simulink model "ControleFF_D_NL"  (R2020b)
settings: Solver=FixedStepAuto  StartTime=0  StopTime=10  FixedStep=1e-3  RelTol=1e-3
values from neighbouring files (symbols this model uses):
  alpha = alpha_vec(l)    [kermani_parameters.m]    (also in teste_controle_nao_linear.m = 1.25)
  Beff = 1    [kermani_parameters.m]    (also in teste_controle_nao_linear.m = 50)
  Fc = Fc_vec(k)    [kermani_parameters.m]    (also in teste_controle_nao_linear.m = 2173.5)
  Fs = Fs_vec(j)    [kermani_parameters.m]    (also in teste_controle_nao_linear.m = 2673.5)
  Jeff = 0.5    [kermani_parameters.m]    (also in teste_controle_nao_linear.m)
  K = (90/12)*(2*pi/60)    (= 0.785398163397)    [kermani_parameters.m]    (also in teste_controle_nao_linear.m)
  Kd = (2*xi*wn*Jeff - Beff)/K    (= 17.8253536263)    [kermani_parameters.m]    (also in teste_controle_nao_linear.m = -44.5633840657)
  Kp = (wn^2*Jeff)/K    (= 143.239448783)    [kermani_parameters.m]    (also in teste_controle_nao_linear.m)
  N = 3    [kermani_parameters.m]    (also in teste_controle_nao_linear.m)
  phi = 43.47    [teste_controle_nao_linear.m]
  r = 1./[231.22*4 139.138 139.138 231.22 231.22]    [kermani_parameters.m]    (also in teste_controle_nao_linear.m)
  sigma0 = sigma0_vec(m)    [kermani_parameters.m]    (also in teste_controle_nao_linear.m = 10000)
  sigma1 = sigma1_vec(n)    [kermani_parameters.m]    (also in teste_controle_nao_linear.m = 1000)
  sigma2 = sigma2_vec(o)    [kermani_parameters.m]    (also in teste_controle_nao_linear.m = 10)
libraries: simulink_extras x21
(part 1 of 14)
settings Model: Creator=Karoline  LastModifiedBy=lunet
settings DataIOCC: ReturnWorkspaceOutputs=off
settings DebuggingCC: ArithmeticOperatorsInVariantConditions=warning
settings SFSimCC: SimUseLocalCustomCode=off  CustomCodeUndefinedFunction=UseInterfaceOnly
settings RTWCC: RTWUseLocalCustomCode=off
settings CodeAppCC: StateflowObjectComments=on

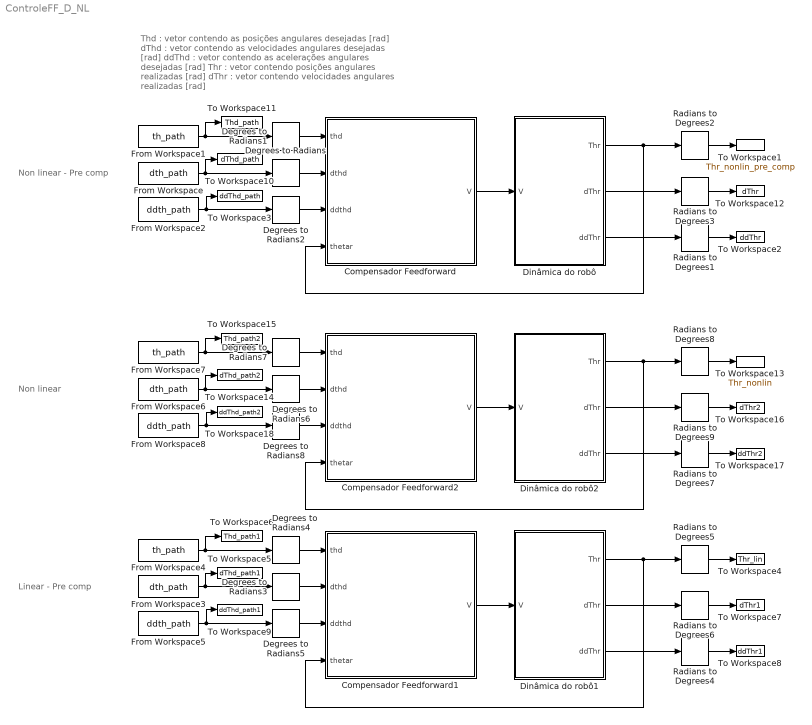
== system ControleFF_D_NL ==
  note: Non linear - Pre comp
  note: Thd : vetor contendo as posições angulares desejadas [rad]
      | dThd : vetor contendo as velocidades angulares desejadas [rad]
      | ddThd : vetor contendo as acelerações angulares desejadas [rad]
      |
      | Thr : vetor contendo posições angulares realizadas [rad]
      | dThr : vetor contendo velocidades angulares realizadas [rad]
  note: Non linear
  note: Linear - Pre comp
  Compensador Feedforward : Subsystem
  Compensador Feedforward1 : Subsystem
  Compensador Feedforward2 : Subsystem
  Degrees to Radians{,1..8} (9 alike) : simulink_extras/Transformations/Degrees to Radians
  Dinâmica do robô : Subsystem
  Dinâmica do robô1 : Subsystem
  Dinâmica do robô2 : Subsystem
  From Workspace : FromWorkspace  VariableName=dth_path
  From Workspace1 : FromWorkspace  VariableName=th_path
  From Workspace2 : FromWorkspace  VariableName=ddth_path
  From Workspace3 : FromWorkspace  VariableName=dth_path
  From Workspace4 : FromWorkspace  VariableName=th_path
  From Workspace5 : FromWorkspace  VariableName=ddth_path
  From Workspace6 : FromWorkspace  VariableName=dth_path
  From Workspace7 : FromWorkspace  VariableName=th_path
  From Workspace8 : FromWorkspace  VariableName=ddth_path
  Radians to Degrees{1..9} (9 alike) : simulink_extras/Transformations/Radians to Degrees
  To Workspace1 : ToWorkspace  VariableName=Thr_nonlin_pre_comp  SaveFormat=Structure With Time  SampleTime=-1
  To Workspace10 : ToWorkspace  VariableName=dThd_path  SaveFormat=Structure With Time  SampleTime=-1
  To Workspace11 : ToWorkspace  VariableName=Thd_path  SaveFormat=Structure With Time  SampleTime=-1
  To Workspace12 : ToWorkspace  VariableName=dThr  SaveFormat=Structure With Time  SampleTime=-1
  To Workspace13 : ToWorkspace  VariableName=Thr_nonlin  SaveFormat=Structure With Time  SampleTime=-1
  To Workspace14 : ToWorkspace  VariableName=dThd_path2  SaveFormat=Structure With Time  SampleTime=-1
  To Workspace15 : ToWorkspace  VariableName=Thd_path2  SaveFormat=Structure With Time  SampleTime=-1
  To Workspace16 : ToWorkspace  VariableName=dThr2  SaveFormat=Structure With Time  SampleTime=-1
  To Workspace17 : ToWorkspace  VariableName=ddThr2  SaveFormat=Structure With Time  SampleTime=-1
  To Workspace18 : ToWorkspace  VariableName=ddThd_path2  SaveFormat=Structure With Time  SampleTime=-1
  To Workspace2 : ToWorkspace  VariableName=ddThr  SaveFormat=Structure With Time  SampleTime=-1
  To Workspace3 : ToWorkspace  VariableName=ddThd_path  SaveFormat=Structure With Time  SampleTime=-1
  To Workspace4 : ToWorkspace  VariableName=Thr_lin  SaveFormat=Structure With Time  SampleTime=-1
  To Workspace5 : ToWorkspace  VariableName=dThd_path1  SaveFormat=Structure With Time  SampleTime=-1
  To Workspace6 : ToWorkspace  VariableName=Thd_path1  SaveFormat=Structure With Time  SampleTime=-1
  To Workspace7 : ToWorkspace  VariableName=dThr1  SaveFormat=Structure With Time  SampleTime=-1
  To Workspace8 : ToWorkspace  VariableName=ddThr1  SaveFormat=Structure With Time  SampleTime=-1
  To Workspace9 : ToWorkspace  VariableName=ddThd_path1  SaveFormat=Structure With Time  SampleTime=-1
  wires:
  Dinâmica do robô/2("dThr ") -> Radians to Degrees3/1
  Compensador Feedforward/1(V) -> Dinâmica do robô/1(V)
  Dinâmica do robô/1(Thr) -> Compensador Feedforward/4(thetar), Radians to Degrees2/1
  From Workspace2/1 -> To Workspace3/1, Degrees to Radians2/1
  Degrees to Radians2/1 -> Compensador Feedforward/3(ddthd)
  From Workspace/1 -> Degrees to Radians/1, To Workspace10/1
  From Workspace1/1 -> Degrees to Radians1/1, To Workspace11/1
  Degrees to Radians1/1 -> Compensador Feedforward/1(thd)
  Degrees to Radians/1 -> Compensador Feedforward/2(dthd)
  Radians to Degrees3/1 -> To Workspace12/1
  Radians to Degrees2/1 -> To Workspace1/1
  Radians to Degrees1/1 -> To Workspace2/1
  Dinâmica do robô/3(ddThr) -> Radians to Degrees1/1
  Degrees to Radians3/1 -> Compensador Feedforward1/2(dthd)
  Radians to Degrees6/1 -> To Workspace7/1
  Radians to Degrees5/1 -> To Workspace4/1
  Radians to Degrees4/1 -> To Workspace8/1
  Dinâmica do robô1/3(ddThr) -> Radians to Degrees4/1
  From Workspace3/1 -> Degrees to Radians3/1, To Workspace5/1
  Dinâmica do robô1/1(Thr) -> Compensador Feedforward1/4(thetar), Radians to Degrees5/1
  From Workspace5/1 -> To Workspace9/1, Degrees to Radians5/1
  From Workspace4/1 -> Degrees to Radians4/1, To Workspace6/1
  Compensador Feedforward1/1(V) -> Dinâmica do robô1/1(V)
  Degrees to Radians5/1 -> Compensador Feedforward1/3(ddthd)
  Degrees to Radians4/1 -> Compensador Feedforward1/1(thd)
  Dinâmica do robô1/2("dThr ") -> Radians to Degrees6/1
  Degrees to Radians6/1 -> Compensador Feedforward2/2(dthd)
  Radians to Degrees9/1 -> To Workspace16/1
  Radians to Degrees8/1 -> To Workspace13/1
  Radians to Degrees7/1 -> To Workspace17/1
  Dinâmica do robô2/3(ddThr) -> Radians to Degrees7/1
  From Workspace6/1 -> Degrees to Radians6/1, To Workspace14/1
  Dinâmica do robô2/1(Thr) -> Compensador Feedforward2/4(thetar), Radians to Degrees8/1
  From Workspace8/1 -> To Workspace18/1, Degrees to Radians8/1
  From Workspace7/1 -> Degrees to Radians7/1, To Workspace15/1
  Compensador Feedforward2/1(V) -> Dinâmica do robô2/1(V)
  Degrees to Radians8/1 -> Compensador Feedforward2/3(ddthd)
  Degrees to Radians7/1 -> Compensador Feedforward2/1(thd)
  Dinâmica do robô2/2("dThr ") -> Radians to Degrees9/1

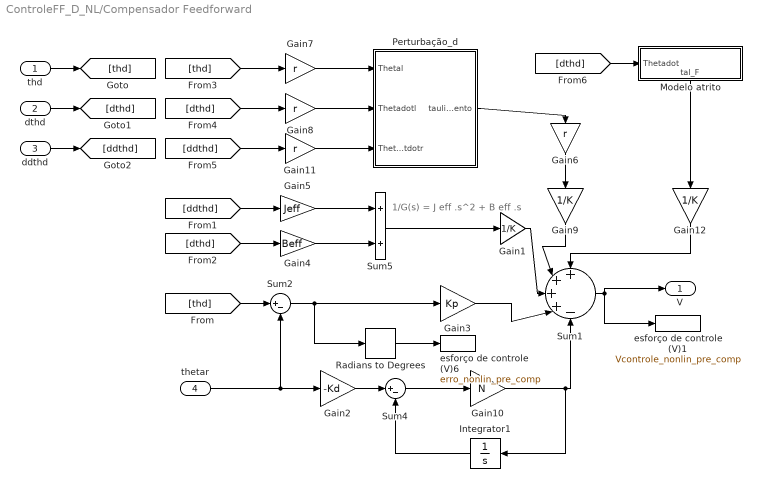
== system ControleFF_D_NL/Compensador Feedforward ==
  note: 1/G(s) = J eff .s^2 + B eff .s
  thd : Inport
  dthd : Inport  Port=2
  ddthd : Inport  Port=3
  thetar : Inport  Port=4
  Gain1 : Gain  Gain=1/K
  Gain10 : Gain  Gain=N
  Gain{6..8,11} (4 alike) : Gain  Gain=r
  Gain12 : Gain  Gain=1/K
  Gain2 : Gain  Gain=-Kd
  Gain3 : Gain  Gain=Kp
  Gain4 : Gain  Gain=Beff
  Gain5 : Gain  Gain=Jeff
  Gain9 : Gain  Gain=1/K
  Integrator1 : Integrator
  Modelo atrito : Subsystem
      settings: PortSchema="{\"entries\":[{\"content\":{\"sides\":[{\"content\":{\"connectorIds\":[\"In1\"]},\"type\":\"ConnectorPlacement.EquallySpacedRectSide\",\"uuid\":\"4cdf76dd-7842-4f53-aa61-23d67f277515\"},{\"content\":{\"connectorIds\":[],\"side\":\"RIGHT\"},\"type\":\"ConnectorPlacement.EquallySpacedRectSide\",\"uuid\":\"e76865b0-8d89-469f-9903-74c23d9bc715\"},{\"content\":{\"connectorIds\":[],\"side\":\"TOP\"},\"type\":\"ConnectorPlacement.EquallySpacedRectSide\",\"uuid\":\"84af05c2-3cf0-417f-8bc5-33473f29c4a4\"},{\"content\":{\"connectorIds\":[\"Out1\"],\"side\":\"BOTTOM\"},\"type\":\"ConnectorPlacement.EquallySpacedRectSide\",\"uuid\":\"8432edb9-61b6-48e7-b184-4a420fe1e6b9\"},{\"content\":{\"connectorIds\":[],\"side\":\"HIDDEN\"},\"type\":\"ConnectorPlacement.EquallySpacedRectSide\",\"uuid\":\"b24fdc73-1a64-48d6-a255-97fbfad7318c\"}]},\"type\":\"ConnectorPlacement.EquallySpacedConnector\",\"uuid\":\"378be7c8-9b7c-4aa3-9a72-c75578af889e\"}],\"packageUris\":[\"http://schema.mathworks.com/mf0/Connector/R2020b\"],\"version\":\"1.0\"}"
  Perturbação_d : Subsystem
  Radians to Degrees : simulink_extras/Transformations/Radians to Degrees
  Sum1 : Sum  Inputs=+|+|+|+|-
  Sum2 : Sum  Inputs=|+-
  Sum4 : Sum  Inputs=|+-
  Sum5 : Sum
  esforço de controle (V)1 : ToWorkspace  VariableName=Vcontrole_nonlin_pre_comp  SaveFormat=Structure With Time  SampleTime=-1
  esforço de controle (V)6 : ToWorkspace  VariableName=erro_nonlin_pre_comp  SaveFormat=Structure With Time  SampleTime=-1
  V : Outport  VectorParamsAs1DForOutWhenUnconnected=off
  wires:
  Gain2/1 -> Sum4/1
  thetar/1 -> Sum2/2, Gain2/1
  Sum4/1 -> Gain10/1
  Integrator1/1 -> Sum4/2
  Gain10/1 -> Sum1/5, Integrator1/1
  Gain4/1 -> Sum5/2
  Gain5/1 -> Sum5/1
  Sum5/1 -> Gain1/1
  Gain8/1 -> Perturbação_d/2(Thetadotl)
  Gain7/1 -> Perturbação_d/1(Thetal)
  [thd] -> Gain7/1
  [dthd] -> Gain8/1
  Perturbação_d/1(tauligamento) -> Gain6/1
  Gain6/1 -> Gain9/1
  Gain9/1 -> Sum1/2
  thd/1 -> [thd]
  [thd] -> Sum2/1
  ddthd/1 -> [ddthd]
  [ddthd] -> Gain5/1
  dthd/1 -> [dthd]
  [dthd] -> Gain4/1
  Gain3/1 -> Sum1/4
  Gain1/1 -> Sum1/3
  Sum1/1 -> V/1, esforço de controle (V)1/1
  Radians to Degrees/1 -> esforço de controle (V)6/1
  Sum2/1 -> Radians to Degrees/1, Gain3/1
  [ddthd] -> Gain11/1
  Gain11/1 -> Perturbação_d/3(Thetadotdotr)
  [dthd] -> Modelo atrito/1(Thetadot)
  Modelo atrito/1(tal_F) -> Gain12/1
  Gain12/1 -> Sum1/1

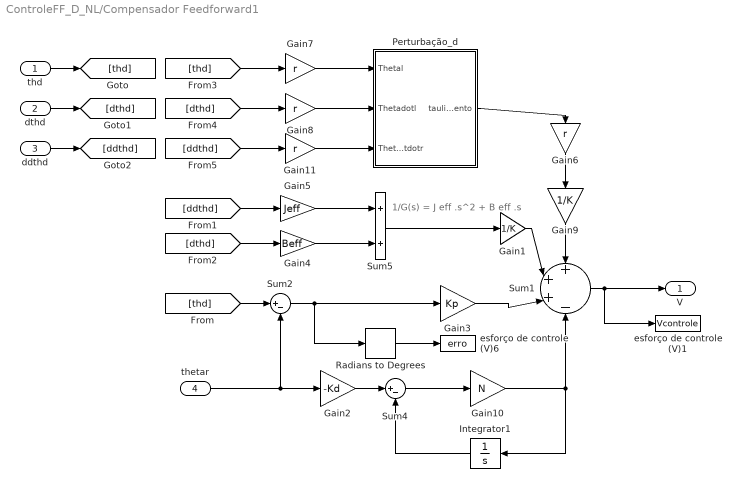
== system ControleFF_D_NL/Compensador Feedforward1 ==
  note: 1/G(s) = J eff .s^2 + B eff .s
  thd : Inport
  dthd : Inport  Port=2
  ddthd : Inport  Port=3
  thetar : Inport  Port=4
  Gain1 : Gain  Gain=1/K
  Gain10 : Gain  Gain=N
  Gain{6..8,11} (4 alike) : Gain  Gain=r
  Gain2 : Gain  Gain=-Kd
  Gain3 : Gain  Gain=Kp
  Gain4 : Gain  Gain=Beff
  Gain5 : Gain  Gain=Jeff
  Gain9 : Gain  Gain=1/K
  Integrator1 : Integrator
  Perturbação_d : Subsystem
  Radians to Degrees : simulink_extras/Transformations/Radians to Degrees
  Sum1 : Sum  Inputs=+|+|+|-
  Sum2 : Sum  Inputs=|+-
  Sum4 : Sum  Inputs=|+-
  Sum5 : Sum
  esforço de controle (V)1 : ToWorkspace  VariableName=Vcontrole  SaveFormat=Structure With Time  SampleTime=-1
  esforço de controle (V)6 : ToWorkspace  VariableName=erro  SaveFormat=Structure With Time  SampleTime=-1
  V : Outport  VectorParamsAs1DForOutWhenUnconnected=off
  wires:
  Gain2/1 -> Sum4/1
  thetar/1 -> Sum2/2, Gain2/1
  Sum4/1 -> Gain10/1
  Integrator1/1 -> Sum4/2
  Gain10/1 -> Sum1/4, Integrator1/1
  Gain4/1 -> Sum5/2
  Gain5/1 -> Sum5/1
  Sum5/1 -> Gain1/1
  Gain8/1 -> Perturbação_d/2(Thetadotl)
  Gain7/1 -> Perturbação_d/1(Thetal)
  [thd] -> Gain7/1
  [dthd] -> Gain8/1
  Perturbação_d/1(tauligamento) -> Gain6/1
  Gain6/1 -> Gain9/1
  Gain9/1 -> Sum1/1
  thd/1 -> [thd]
  [thd] -> Sum2/1
  ddthd/1 -> [ddthd]
  [ddthd] -> Gain5/1
  dthd/1 -> [dthd]
  [dthd] -> Gain4/1
  Gain3/1 -> Sum1/3
  Gain1/1 -> Sum1/2
  Sum1/1 -> esforço de controle (V)1/1, V/1
  Radians to Degrees/1 -> esforço de controle (V)6/1
  Sum2/1 -> Radians to Degrees/1, Gain3/1
  [ddthd] -> Gain11/1
  Gain11/1 -> Perturbação_d/3(Thetadotdotr)

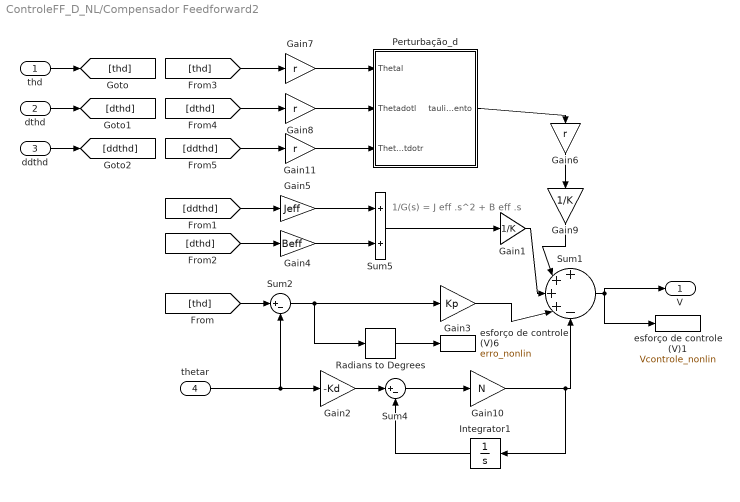
== system ControleFF_D_NL/Compensador Feedforward2 ==
  note: 1/G(s) = J eff .s^2 + B eff .s
  thd : Inport
  dthd : Inport  Port=2
  ddthd : Inport  Port=3
  thetar : Inport  Port=4
  Gain1 : Gain  Gain=1/K
  Gain10 : Gain  Gain=N
  Gain{6..8,11} (4 alike) : Gain  Gain=r
  Gain2 : Gain  Gain=-Kd
  Gain3 : Gain  Gain=Kp
  Gain4 : Gain  Gain=Beff
  Gain5 : Gain  Gain=Jeff
  Gain9 : Gain  Gain=1/K
  Integrator1 : Integrator
  Perturbação_d : Subsystem
  Radians to Degrees : simulink_extras/Transformations/Radians to Degrees
  Sum1 : Sum  Inputs=+|+|+|+|-
  Sum2 : Sum  Inputs=|+-
  Sum4 : Sum  Inputs=|+-
  Sum5 : Sum
  esforço de controle (V)1 : ToWorkspace  VariableName=Vcontrole_nonlin  SaveFormat=Structure With Time  SampleTime=-1
  esforço de controle (V)6 : ToWorkspace  VariableName=erro_nonlin  SaveFormat=Structure With Time  SampleTime=-1
  V : Outport  VectorParamsAs1DForOutWhenUnconnected=off
  wires:
  Gain2/1 -> Sum4/1
  thetar/1 -> Sum2/2, Gain2/1
  Sum4/1 -> Gain10/1
  Integrator1/1 -> Sum4/2
  Gain10/1 -> Sum1/5, Integrator1/1
  Gain4/1 -> Sum5/2
  Gain5/1 -> Sum5/1
  Sum5/1 -> Gain1/1
  Gain8/1 -> Perturbação_d/2(Thetadotl)
  Gain7/1 -> Perturbação_d/1(Thetal)
  [thd] -> Gain7/1
  [dthd] -> Gain8/1
  Perturbação_d/1(tauligamento) -> Gain6/1
  Gain6/1 -> Gain9/1
  Gain9/1 -> Sum1/2
  thd/1 -> [thd]
  [thd] -> Sum2/1
  ddthd/1 -> [ddthd]
  [ddthd] -> Gain5/1
  dthd/1 -> [dthd]
  [dthd] -> Gain4/1
  Gain3/1 -> Sum1/4
  Gain1/1 -> Sum1/3
  Sum1/1 -> V/1, esforço de controle (V)1/1
  Radians to Degrees/1 -> esforço de controle (V)6/1
  Sum2/1 -> Radians to Degrees/1, Gain3/1
  [ddthd] -> Gain11/1
  Gain11/1 -> Perturbação_d/3(Thetadotdotr)

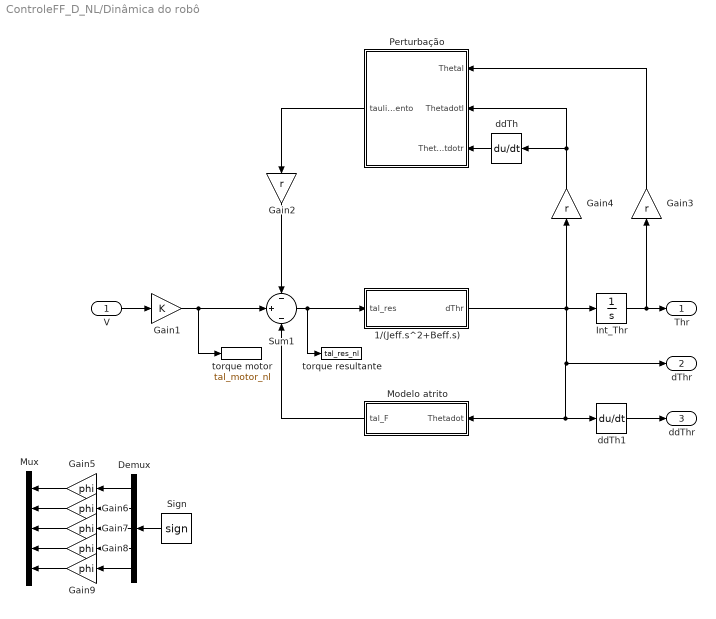
== system ControleFF_D_NL/Dinâmica do robô ==
  V : Inport
  1/(Jeff.s^2+Beff.s) : Subsystem
  Demux : Demux  Outputs=5
  Gain1 : Gain  Gain=K
  Gain2 : Gain  Gain=r
  Gain3 : Gain  Gain=r
  Gain4 : Gain  Gain=r
  Gain{5..9} (5 alike) : Gain  Gain=phi
  Int_Thr : Integrator  Tag=Int_Thr  InitialCondition=[0 0 0 0 0]
  Modelo atrito : Subsystem
  Mux : Mux  Inputs=5
  Perturbação : Subsystem
  Sign : Signum
  Sum1 : Sum  Inputs=-|+|-
  ddTh : Derivative
  ddTh1 : Derivative
  torque motor : ToWorkspace  VariableName=tal_motor_nl  SaveFormat=Structure With Time  SampleTime=-1
  torque resultante : ToWorkspace  VariableName=tal_res_nl  SaveFormat=Structure With Time  SampleTime=-1
  Thr : Outport  VectorParamsAs1DForOutWhenUnconnected=off
  "dThr " : Outport  Port=2  VectorParamsAs1DForOutWhenUnconnected=off
  ddThr : Outport  Port=3  VectorParamsAs1DForOutWhenUnconnected=off
  wires:
  Perturbação/1(tauligamento) -> Gain2/1
  Gain1/1 -> torque motor/1, Sum1/2
  Int_Thr/1 -> Thr/1, Gain3/1
  V/1 -> Gain1/1
  Gain2/1 -> Sum1/1
  ddTh/1 -> Perturbação/3(Thetadotdotr)
  Gain3/1 -> Perturbação/1(Thetal)
  Gain4/1 -> ddTh/1, Perturbação/2(Thetadotl)
  Sum1/1 -> torque resultante/1, 1/(Jeff.s^2+Beff.s)/1(tal_res)
  ddTh1/1 -> ddThr/1
  Sign/1 -> Demux/1
  Demux/1 -> Gain5/1
  Gain5/1 -> Mux/1
  Demux/2 -> Gain6/1
  Demux/3 -> Gain7/1
  Demux/4 -> Gain8/1
  Demux/5 -> Gain9/1
  Gain6/1 -> Mux/2
  Gain7/1 -> Mux/3
  Gain8/1 -> Mux/4
  Gain9/1 -> Mux/5
  1/(Jeff.s^2+Beff.s)/1(dThr) -> Modelo atrito/1(Thetadot), ddTh1/1, "dThr "/1, Gain4/1, Int_Thr/1
  Modelo atrito/1(tal_F) -> Sum1/3

== system ControleFF_D_NL/Dinâmica do robô1 ==
  V : Inport
  1/(Jeff.s^2+Beff.s) : Subsystem
  Demux : Demux  Outputs=5
  Gain1 : Gain  Gain=K
  Gain2 : Gain  Gain=r
  Gain3 : Gain  Gain=r
  Gain4 : Gain  Gain=r
  Gain{5..9} (5 alike) : Gain  Gain=phi
  Int_Thr : Integrator  Tag=Int_Thr  InitialCondition=[0 0 0 0 0]
  Mux : Mux  Inputs=5
  Perturbação : Subsystem
  Scope1 : Scope
  Sign : Signum
  Sum1 : Sum  Inputs=-+|
  ddTh : Derivative
  ddTh1 : Derivative
  torque motor : ToWorkspace  VariableName=tal_motor  SaveFormat=Structure With Time  SampleTime=-1
  torque resultante : ToWorkspace  VariableName=tal_res  SaveFormat=Structure With Time  SampleTime=-1
  Thr : Outport  VectorParamsAs1DForOutWhenUnconnected=off
  "dThr " : Outport  Port=2  VectorParamsAs1DForOutWhenUnconnected=off
  ddThr : Outport  Port=3  VectorParamsAs1DForOutWhenUnconnected=off
  wires:
  Perturbação/1(tauligamento) -> Gain2/1
  Gain1/1 -> torque motor/1, Sum1/2
  Int_Thr/1 -> Thr/1, Scope1/1, Gain3/1
  V/1 -> Gain1/1
  Gain2/1 -> Sum1/1
  ddTh/1 -> Perturbação/3(Thetadotdotr)
  Gain3/1 -> Perturbação/1(Thetal)
  Gain4/1 -> ddTh/1, Perturbação/2(Thetadotl)
  Sum1/1 -> torque resultante/1, 1/(Jeff.s^2+Beff.s)/1(tal_res)
  ddTh1/1 -> ddThr/1
  Sign/1 -> Demux/1
  Demux/1 -> Gain5/1
  Gain5/1 -> Mux/1
  Demux/2 -> Gain6/1
  Demux/3 -> Gain7/1
  Demux/4 -> Gain8/1
  Demux/5 -> Gain9/1
  Gain6/1 -> Mux/2
  Gain7/1 -> Mux/3
  Gain8/1 -> Mux/4
  Gain9/1 -> Mux/5
  1/(Jeff.s^2+Beff.s)/1(dThr) -> ddTh1/1, "dThr "/1, Gain4/1, Int_Thr/1

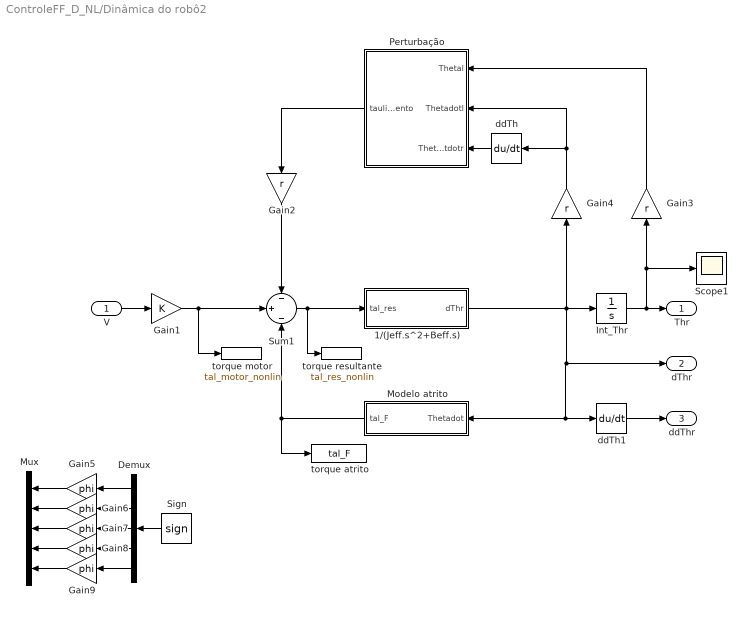
== system ControleFF_D_NL/Dinâmica do robô2 ==
  V : Inport
  1/(Jeff.s^2+Beff.s) : Subsystem
  Demux : Demux  Outputs=5
  Gain1 : Gain  Gain=K
  Gain2 : Gain  Gain=r
  Gain3 : Gain  Gain=r
  Gain4 : Gain  Gain=r
  Gain{5..9} (5 alike) : Gain  Gain=phi
  Int_Thr : Integrator  Tag=Int_Thr  InitialCondition=[0 0 0 0 0]
  Modelo atrito : Subsystem
  Mux : Mux  Inputs=5
  Perturbação : Subsystem
  Scope1 : Scope
  Sign : Signum
  Sum1 : Sum  Inputs=-|+|-
  ddTh : Derivative
  ddTh1 : Derivative
  torque atrito : ToWorkspace  VariableName=tal_F  SaveFormat=Structure With Time  SampleTime=-1
  torque motor : ToWorkspace  VariableName=tal_motor_nonlin  SaveFormat=Structure With Time  SampleTime=-1
  torque resultante : ToWorkspace  VariableName=tal_res_nonlin  SaveFormat=Structure With Time  SampleTime=-1
  Thr : Outport  VectorParamsAs1DForOutWhenUnconnected=off
  "dThr " : Outport  Port=2  VectorParamsAs1DForOutWhenUnconnected=off
  ddThr : Outport  Port=3  VectorParamsAs1DForOutWhenUnconnected=off
  wires:
  Perturbação/1(tauligamento) -> Gain2/1
  Gain1/1 -> torque motor/1, Sum1/2
  Int_Thr/1 -> Thr/1, Scope1/1, Gain3/1
  V/1 -> Gain1/1
  Gain2/1 -> Sum1/1
  ddTh/1 -> Perturbação/3(Thetadotdotr)
  Gain3/1 -> Perturbação/1(Thetal)
  Gain4/1 -> ddTh/1, Perturbação/2(Thetadotl)
  Sum1/1 -> torque resultante/1, 1/(Jeff.s^2+Beff.s)/1(tal_res)
  ddTh1/1 -> ddThr/1
  Sign/1 -> Demux/1
  Demux/1 -> Gain5/1
  Gain5/1 -> Mux/1
  Demux/2 -> Gain6/1
  Demux/3 -> Gain7/1
  Demux/4 -> Gain8/1
  Demux/5 -> Gain9/1
  Gain6/1 -> Mux/2
  Gain7/1 -> Mux/3
  Gain8/1 -> Mux/4
  Gain9/1 -> Mux/5
  1/(Jeff.s^2+Beff.s)/1(dThr) -> Modelo atrito/1(Thetadot), ddTh1/1, "dThr "/1, Gain4/1, Int_Thr/1
  Modelo atrito/1(tal_F) -> Sum1/3, torque atrito/1

== system ControleFF_D_NL/Compensador Feedforward/Modelo atrito ==
  note: z
  note: zdot
  Thetadot : Inport
  Abs : Abs
  Add : Sum  Inputs=+++
  Divide : Product  Inputs=*/*
  Integrator : Integrator
  Sigma0 : Gain  Gain=sigma0
  Sigma1 : Gain  Gain=sigma1
  Sigma2 : Gain  Gain=sigma2
  Sum : Sum  Inputs=|+-
  s_Thetadot : Subsystem
      settings: PortSchema="{\"entries\":[{\"content\":{\"sides\":[{\"content\":{\"connectorIds\":[]},\"type\":\"ConnectorPlacement.EquallySpacedRectSide\",\"uuid\":\"4c4b190b-c928-4253-93d1-fd2ae137e0ab\"},{\"content\":{\"connectorIds\":[\"Out1\"],\"side\":\"RIGHT\"},\"type\":\"ConnectorPlacement.EquallySpacedRectSide\",\"uuid\":\"6a4109ad-b0a7-44dc-94f8-84112378c3da\"},{\"content\":{\"connectorIds\":[\"In1\"],\"side\":\"TOP\"},\"type\":\"ConnectorPlacement.EquallySpacedRectSide\",\"uuid\":\"364d9b06-17df-4fa5-ae25-87ed6816814d\"},{\"content\":{\"connectorIds\":[],\"side\":\"HIDDEN\"},\"type\":\"ConnectorPlacement.EquallySpacedRectSide\",\"uuid\":\"e93aa933-b8be-40f2-a8c0-ee27516241e6\"}]},\"type\":\"ConnectorPlacement.EquallySpacedConnector\",\"uuid\":\"c598e9c2-b687-45ab-b3d0-f2b281a49fb7\"}],\"packageUris\":[\"http://schema.mathworks.com/mf0/Connector/R2020b\"],\"version\":\"1.0\"}"
  tal_F : Outport
  wires:
  Sigma0/1 -> Divide/3, Add/3
  Sigma1/1 -> Add/2
  Divide/1 -> Sum/2
  Abs/1 -> s_Thetadot/1(|Thetadot|), Divide/1
  s_Thetadot/1(s_Thetadot) -> Divide/2
  Sum/1 -> Sigma1/1, Integrator/1
  Thetadot/1 -> Sigma2/1, Sum/1, Abs/1
  Sigma2/1 -> Add/1
  Integrator/1 -> Sigma0/1
  Add/1 -> tal_F/1

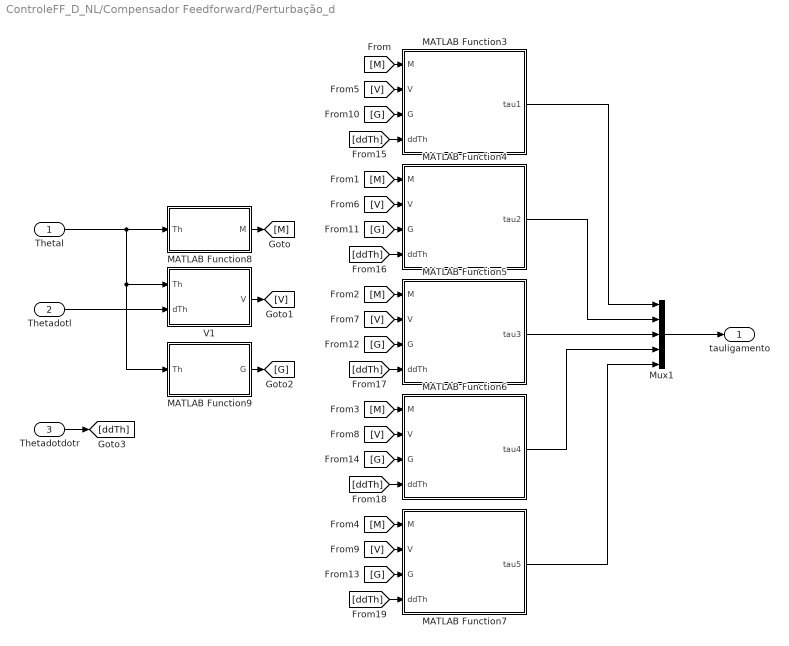
== system ControleFF_D_NL/Compensador Feedforward/Perturbação_d ==
  Thetal : Inport
  Thetadotl : Inport  Port=2
  Thetadotdotr : Inport  Port=3
  MATLAB Function3 : MATLAB Function  TreatAsAtomicUnit=on
  MATLAB Function4 : MATLAB Function  TreatAsAtomicUnit=on
  MATLAB Function5 : MATLAB Function  TreatAsAtomicUnit=on
  MATLAB Function6 : MATLAB Function  TreatAsAtomicUnit=on
  MATLAB Function7 : MATLAB Function  TreatAsAtomicUnit=on
  MATLAB Function8 : MATLAB Function  TreatAsAtomicUnit=on
  MATLAB Function9 : MATLAB Function  TreatAsAtomicUnit=on
  Mux1 : Mux  Inputs=5
  V1 : MATLAB Function  TreatAsAtomicUnit=on
  tauligamento : Outport  VectorParamsAs1DForOutWhenUnconnected=off
  wires:
  [G] -> MATLAB Function6/3(G)
  MATLAB Function8/1(M) -> [M]
  [M] -> MATLAB Function6/1(M)
  [M] -> MATLAB Function4/1(M)
  [M] -> MATLAB Function3/1(M)
  Thetal/1 -> MATLAB Function8/1(Th), MATLAB Function9/1(Th), V1/1(Th)
  [ddTh] -> MATLAB Function5/4(ddTh)
  [V] -> MATLAB Function3/2(V)
  [ddTh] -> MATLAB Function3/4(ddTh)
  [G] -> MATLAB Function7/3(G)
  [ddTh] -> MATLAB Function6/4(ddTh)
  [V] -> MATLAB Function6/2(V)
  Thetadotl/1 -> V1/2(dTh)
  [G] -> MATLAB Function5/3(G)
  [G] -> MATLAB Function3/3(G)
  [G] -> MATLAB Function4/3(G)
  MATLAB Function9/1(G) -> [G]
  [V] -> MATLAB Function7/2(V)
  [ddTh] -> MATLAB Function4/4(ddTh)
  [V] -> MATLAB Function5/2(V)
  [V] -> MATLAB Function4/2(V)
  V1/1(V) -> [V]
  [M] -> MATLAB Function7/1(M)
  [M] -> MATLAB Function5/1(M)
  [ddTh] -> MATLAB Function7/4(ddTh)
  Mux1/1 -> tauligamento/1
  MATLAB Function3/1(tau1) -> Mux1/1
  MATLAB Function4/1(tau2) -> Mux1/2
  MATLAB Function5/1(tau3) -> Mux1/3
  MATLAB Function6/1(tau4) -> Mux1/4
  MATLAB Function7/1(tau5) -> Mux1/5
  Thetadotdotr/1 -> [ddTh]

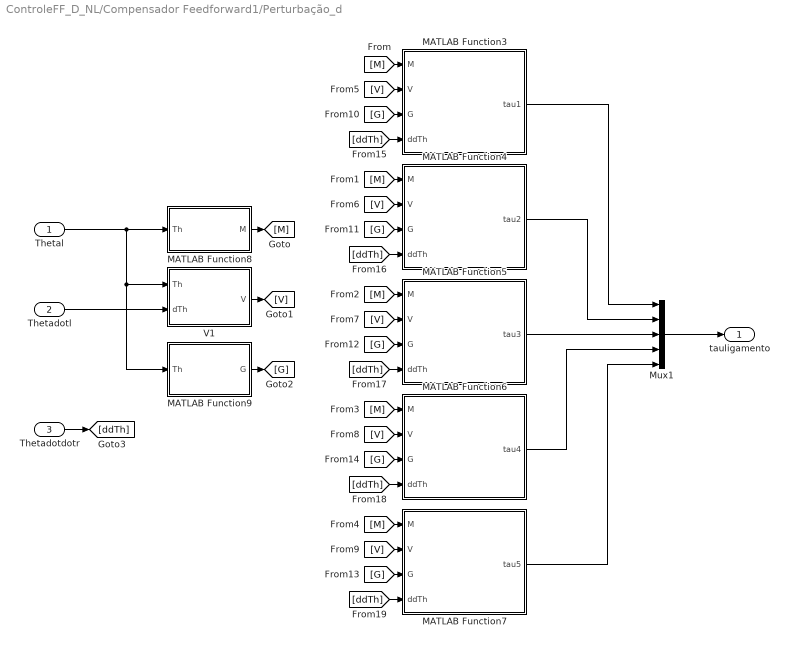
== system ControleFF_D_NL/Compensador Feedforward1/Perturbação_d ==
  Thetal : Inport
  Thetadotl : Inport  Port=2
  Thetadotdotr : Inport  Port=3
  MATLAB Function3 : MATLAB Function  TreatAsAtomicUnit=on
  MATLAB Function4 : MATLAB Function  TreatAsAtomicUnit=on
  MATLAB Function5 : MATLAB Function  TreatAsAtomicUnit=on
  MATLAB Function6 : MATLAB Function  TreatAsAtomicUnit=on
  MATLAB Function7 : MATLAB Function  TreatAsAtomicUnit=on
  MATLAB Function8 : MATLAB Function  TreatAsAtomicUnit=on
  MATLAB Function9 : MATLAB Function  TreatAsAtomicUnit=on
  Mux1 : Mux  Inputs=5
  V1 : MATLAB Function  TreatAsAtomicUnit=on
  tauligamento : Outport  VectorParamsAs1DForOutWhenUnconnected=off
  wires:
  [G] -> MATLAB Function6/3(G)
  MATLAB Function8/1(M) -> [M]
  [M] -> MATLAB Function6/1(M)
  [M] -> MATLAB Function4/1(M)
  [M] -> MATLAB Function3/1(M)
  Thetal/1 -> MATLAB Function8/1(Th), MATLAB Function9/1(Th), V1/1(Th)
  [ddTh] -> MATLAB Function5/4(ddTh)
  [V] -> MATLAB Function3/2(V)
  [ddTh] -> MATLAB Function3/4(ddTh)
  [G] -> MATLAB Function7/3(G)
  [ddTh] -> MATLAB Function6/4(ddTh)
  [V] -> MATLAB Function6/2(V)
  Thetadotl/1 -> V1/2(dTh)
  [G] -> MATLAB Function5/3(G)
  [G] -> MATLAB Function3/3(G)
  [G] -> MATLAB Function4/3(G)
  MATLAB Function9/1(G) -> [G]
  [V] -> MATLAB Function7/2(V)
  [ddTh] -> MATLAB Function4/4(ddTh)
  [V] -> MATLAB Function5/2(V)
  [V] -> MATLAB Function4/2(V)
  V1/1(V) -> [V]
  [M] -> MATLAB Function7/1(M)
  [M] -> MATLAB Function5/1(M)
  [ddTh] -> MATLAB Function7/4(ddTh)
  Mux1/1 -> tauligamento/1
  MATLAB Function3/1(tau1) -> Mux1/1
  MATLAB Function4/1(tau2) -> Mux1/2
  MATLAB Function5/1(tau3) -> Mux1/3
  MATLAB Function6/1(tau4) -> Mux1/4
  MATLAB Function7/1(tau5) -> Mux1/5
  Thetadotdotr/1 -> [ddTh]

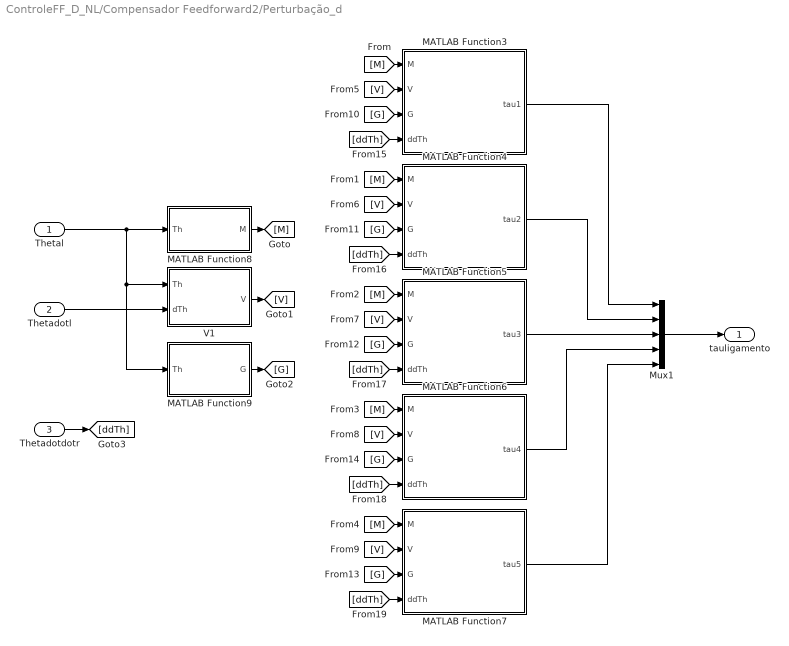
== system ControleFF_D_NL/Compensador Feedforward2/Perturbação_d ==
  Thetal : Inport
  Thetadotl : Inport  Port=2
  Thetadotdotr : Inport  Port=3
  MATLAB Function3 : MATLAB Function  TreatAsAtomicUnit=on
  MATLAB Function4 : MATLAB Function  TreatAsAtomicUnit=on
  MATLAB Function5 : MATLAB Function  TreatAsAtomicUnit=on
  MATLAB Function6 : MATLAB Function  TreatAsAtomicUnit=on
  MATLAB Function7 : MATLAB Function  TreatAsAtomicUnit=on
  MATLAB Function8 : MATLAB Function  TreatAsAtomicUnit=on
  MATLAB Function9 : MATLAB Function  TreatAsAtomicUnit=on
  Mux1 : Mux  Inputs=5
  V1 : MATLAB Function  TreatAsAtomicUnit=on
  tauligamento : Outport  VectorParamsAs1DForOutWhenUnconnected=off
  wires:
  [G] -> MATLAB Function6/3(G)
  MATLAB Function8/1(M) -> [M]
  [M] -> MATLAB Function6/1(M)
  [M] -> MATLAB Function4/1(M)
  [M] -> MATLAB Function3/1(M)
  Thetal/1 -> MATLAB Function8/1(Th), MATLAB Function9/1(Th), V1/1(Th)
  [ddTh] -> MATLAB Function5/4(ddTh)
  [V] -> MATLAB Function3/2(V)
  [ddTh] -> MATLAB Function3/4(ddTh)
  [G] -> MATLAB Function7/3(G)
  [ddTh] -> MATLAB Function6/4(ddTh)
  [V] -> MATLAB Function6/2(V)
  Thetadotl/1 -> V1/2(dTh)
  [G] -> MATLAB Function5/3(G)
  [G] -> MATLAB Function3/3(G)
  [G] -> MATLAB Function4/3(G)
  MATLAB Function9/1(G) -> [G]
  [V] -> MATLAB Function7/2(V)
  [ddTh] -> MATLAB Function4/4(ddTh)
  [V] -> MATLAB Function5/2(V)
  [V] -> MATLAB Function4/2(V)
  V1/1(V) -> [V]
  [M] -> MATLAB Function7/1(M)
  [M] -> MATLAB Function5/1(M)
  [ddTh] -> MATLAB Function7/4(ddTh)
  Mux1/1 -> tauligamento/1
  MATLAB Function3/1(tau1) -> Mux1/1
  MATLAB Function4/1(tau2) -> Mux1/2
  MATLAB Function5/1(tau3) -> Mux1/3
  MATLAB Function6/1(tau4) -> Mux1/4
  MATLAB Function7/1(tau5) -> Mux1/5
  Thetadotdotr/1 -> [ddTh]

== system ControleFF_D_NL/Dinâmica do robô/1//(Jeff.s^2+Beff.s) ==
  tal_res : Inport
  Demux1 : Demux  Outputs=5
  Modelo Juntas{1..5} (5 alike) : TransferFcn  Denominator=[Jeff Beff]
  Mux1 : Mux  Inputs=5
  dThr : Outport
  wires:
  Modelo Juntas5/1 -> Mux1/1
  Demux1/1 -> Modelo Juntas5/1
  Mux1/1 -> dThr/1
  tal_res/1 -> Demux1/1
  Demux1/2 -> Modelo Juntas1/1
  Modelo Juntas1/1 -> Mux1/2
  Demux1/5 -> Modelo Juntas4/1
  Demux1/4 -> Modelo Juntas3/1
  Demux1/3 -> Modelo Juntas2/1
  Modelo Juntas2/1 -> Mux1/3
  Modelo Juntas3/1 -> Mux1/4
  Modelo Juntas4/1 -> Mux1/5

== system ControleFF_D_NL/Dinâmica do robô/Modelo atrito ==
  note: z
  note: zdot
  Thetadot : Inport
  Abs : Abs
  Add : Sum  Inputs=+++
  Divide : Product  Inputs=*/*
  Integrator : Integrator
  Sigma0 : Gain  Gain=sigma0
  Sigma1 : Gain  Gain=sigma1
  Sigma2 : Gain  Gain=sigma2
  Sum : Sum  Inputs=|+-
  s_Thetadot : Subsystem
      settings: PortSchema="{\"entries\":[{\"content\":{\"sides\":[{\"content\":{\"connectorIds\":[]},\"type\":\"ConnectorPlacement.EquallySpacedRectSide\",\"uuid\":\"4c4b190b-c928-4253-93d1-fd2ae137e0ab\"},{\"content\":{\"connectorIds\":[\"Out1\"],\"side\":\"RIGHT\"},\"type\":\"ConnectorPlacement.EquallySpacedRectSide\",\"uuid\":\"6a4109ad-b0a7-44dc-94f8-84112378c3da\"},{\"content\":{\"connectorIds\":[\"In1\"],\"side\":\"TOP\"},\"type\":\"ConnectorPlacement.EquallySpacedRectSide\",\"uuid\":\"364d9b06-17df-4fa5-ae25-87ed6816814d\"},{\"content\":{\"connectorIds\":[],\"side\":\"HIDDEN\"},\"type\":\"ConnectorPlacement.EquallySpacedRectSide\",\"uuid\":\"e93aa933-b8be-40f2-a8c0-ee27516241e6\"}]},\"type\":\"ConnectorPlacement.EquallySpacedConnector\",\"uuid\":\"c598e9c2-b687-45ab-b3d0-f2b281a49fb7\"}],\"packageUris\":[\"http://schema.mathworks.com/mf0/Connector/R2020b\"],\"version\":\"1.0\"}"
  tal_F : Outport
  wires:
  Sigma0/1 -> Divide/3, Add/3
  Sigma1/1 -> Add/2
  Divide/1 -> Sum/2
  Abs/1 -> s_Thetadot/1(|Thetadot|), Divide/1
  s_Thetadot/1(s_Thetadot) -> Divide/2
  Sum/1 -> Sigma1/1, Integrator/1
  Thetadot/1 -> Sigma2/1, Sum/1, Abs/1
  Sigma2/1 -> Add/1
  Integrator/1 -> Sigma0/1
  Add/1 -> tal_F/1

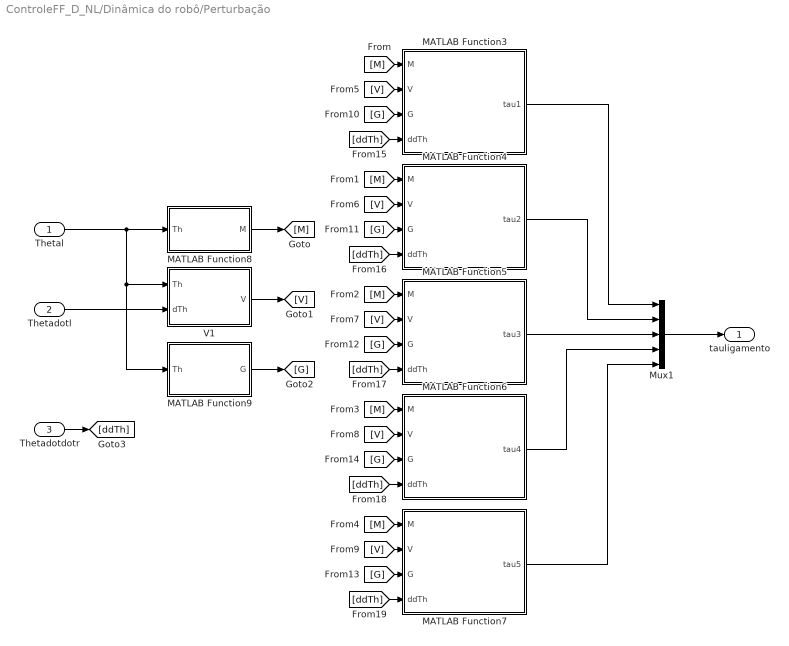
== system ControleFF_D_NL/Dinâmica do robô/Perturbação ==
  Thetal : Inport
  Thetadotl : Inport  Port=2
  Thetadotdotr : Inport  Port=3
  MATLAB Function3 : MATLAB Function  TreatAsAtomicUnit=on
  MATLAB Function4 : MATLAB Function  TreatAsAtomicUnit=on
  MATLAB Function5 : MATLAB Function  TreatAsAtomicUnit=on
  MATLAB Function6 : MATLAB Function  TreatAsAtomicUnit=on
  MATLAB Function7 : MATLAB Function  TreatAsAtomicUnit=on
  MATLAB Function8 : MATLAB Function  TreatAsAtomicUnit=on
  MATLAB Function9 : MATLAB Function  TreatAsAtomicUnit=on
  Mux1 : Mux  Inputs=5
  V1 : MATLAB Function  TreatAsAtomicUnit=on
  tauligamento : Outport  VectorParamsAs1DForOutWhenUnconnected=off
  wires:
  [G] -> MATLAB Function6/3(G)
  MATLAB Function8/1(M) -> [M]
  [M] -> MATLAB Function6/1(M)
  [M] -> MATLAB Function4/1(M)
  [M] -> MATLAB Function3/1(M)
  Thetal/1 -> MATLAB Function8/1(Th), MATLAB Function9/1(Th), V1/1(Th)
  [ddTh] -> MATLAB Function5/4(ddTh)
  [V] -> MATLAB Function3/2(V)
  [ddTh] -> MATLAB Function3/4(ddTh)
  [G] -> MATLAB Function7/3(G)
  [ddTh] -> MATLAB Function6/4(ddTh)
  [V] -> MATLAB Function6/2(V)
  Thetadotl/1 -> V1/2(dTh)
  [G] -> MATLAB Function5/3(G)
  [G] -> MATLAB Function3/3(G)
  [G] -> MATLAB Function4/3(G)
  MATLAB Function9/1(G) -> [G]
  [V] -> MATLAB Function7/2(V)
  [ddTh] -> MATLAB Function4/4(ddTh)
  [V] -> MATLAB Function5/2(V)
  [V] -> MATLAB Function4/2(V)
  V1/1(V) -> [V]
  [M] -> MATLAB Function7/1(M)
  [M] -> MATLAB Function5/1(M)
  [ddTh] -> MATLAB Function7/4(ddTh)
  Mux1/1 -> tauligamento/1
  MATLAB Function3/1(tau1) -> Mux1/1
  MATLAB Function4/1(tau2) -> Mux1/2
  MATLAB Function5/1(tau3) -> Mux1/3
  MATLAB Function6/1(tau4) -> Mux1/4
  MATLAB Function7/1(tau5) -> Mux1/5
  Thetadotdotr/1 -> [ddTh]

== system ControleFF_D_NL/Dinâmica do robô1/1//(Jeff.s^2+Beff.s) ==
  tal_res : Inport
  Demux1 : Demux  Outputs=5
  Modelo Juntas{1..5} (5 alike) : TransferFcn  Denominator=[Jeff Beff]
  Mux1 : Mux  Inputs=5
  dThr : Outport
  wires:
  Modelo Juntas5/1 -> Mux1/1
  Demux1/1 -> Modelo Juntas5/1
  Mux1/1 -> dThr/1
  tal_res/1 -> Demux1/1
  Demux1/2 -> Modelo Juntas1/1
  Modelo Juntas1/1 -> Mux1/2
  Demux1/5 -> Modelo Juntas4/1
  Demux1/4 -> Modelo Juntas3/1
  Demux1/3 -> Modelo Juntas2/1
  Modelo Juntas2/1 -> Mux1/3
  Modelo Juntas3/1 -> Mux1/4
  Modelo Juntas4/1 -> Mux1/5

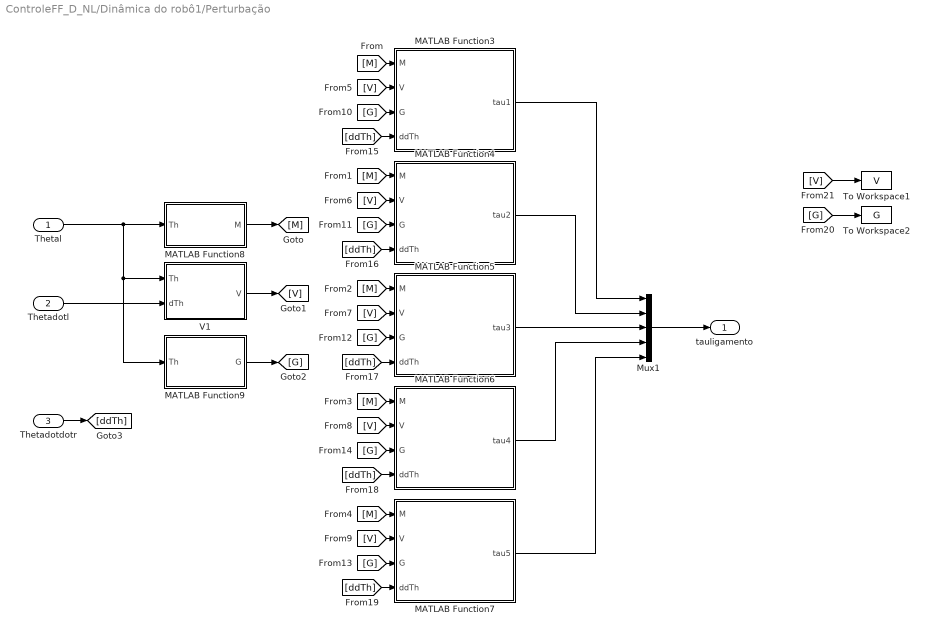
== system ControleFF_D_NL/Dinâmica do robô1/Perturbação ==
  Thetal : Inport
  Thetadotl : Inport  Port=2
  Thetadotdotr : Inport  Port=3
  MATLAB Function3 : MATLAB Function  TreatAsAtomicUnit=on
  MATLAB Function4 : MATLAB Function  TreatAsAtomicUnit=on
  MATLAB Function5 : MATLAB Function  TreatAsAtomicUnit=on
  MATLAB Function6 : MATLAB Function  TreatAsAtomicUnit=on
  MATLAB Function7 : MATLAB Function  TreatAsAtomicUnit=on
  MATLAB Function8 : MATLAB Function  TreatAsAtomicUnit=on
  MATLAB Function9 : MATLAB Function  TreatAsAtomicUnit=on
  Mux1 : Mux  Inputs=5
  To Workspace1 : ToWorkspace  VariableName=V  SaveFormat=Structure With Time  SampleTime=-1
  To Workspace2 : ToWorkspace  VariableName=G  SaveFormat=Structure With Time  SampleTime=-1
  V1 : MATLAB Function  TreatAsAtomicUnit=on
  tauligamento : Outport  VectorParamsAs1DForOutWhenUnconnected=off
  wires:
  [G] -> MATLAB Function6/3(G)
  MATLAB Function8/1(M) -> [M]
  [M] -> MATLAB Function6/1(M)
  [M] -> MATLAB Function4/1(M)
  [M] -> MATLAB Function3/1(M)
  Thetal/1 -> MATLAB Function8/1(Th), MATLAB Function9/1(Th), V1/1(Th)
  [ddTh] -> MATLAB Function5/4(ddTh)
  [V] -> MATLAB Function3/2(V)
  [ddTh] -> MATLAB Function3/4(ddTh)
  [G] -> MATLAB Function7/3(G)
  [ddTh] -> MATLAB Function6/4(ddTh)
  [V] -> MATLAB Function6/2(V)
  Thetadotl/1 -> V1/2(dTh)
  [G] -> MATLAB Function5/3(G)
  [G] -> MATLAB Function3/3(G)
  [G] -> MATLAB Function4/3(G)
  MATLAB Function9/1(G) -> [G]
  [V] -> MATLAB Function7/2(V)
  [ddTh] -> MATLAB Function4/4(ddTh)
  [V] -> MATLAB Function5/2(V)
  [V] -> MATLAB Function4/2(V)
  V1/1(V) -> [V]
  [M] -> MATLAB Function7/1(M)
  [M] -> MATLAB Function5/1(M)
  [ddTh] -> MATLAB Function7/4(ddTh)
  Mux1/1 -> tauligamento/1
  MATLAB Function3/1(tau1) -> Mux1/1
  MATLAB Function4/1(tau2) -> Mux1/2
  MATLAB Function5/1(tau3) -> Mux1/3
  MATLAB Function6/1(tau4) -> Mux1/4
  MATLAB Function7/1(tau5) -> Mux1/5
  Thetadotdotr/1 -> [ddTh]
  [G] -> To Workspace2/1
  [V] -> To Workspace1/1

== system ControleFF_D_NL/Dinâmica do robô2/1//(Jeff.s^2+Beff.s) ==
  tal_res : Inport
  Demux1 : Demux  Outputs=5
  Modelo Juntas{1..5} (5 alike) : TransferFcn  Denominator=[Jeff Beff]
  Mux1 : Mux  Inputs=5
  dThr : Outport
  wires:
  Modelo Juntas5/1 -> Mux1/1
  Demux1/1 -> Modelo Juntas5/1
  Mux1/1 -> dThr/1
  tal_res/1 -> Demux1/1
  Demux1/2 -> Modelo Juntas1/1
  Modelo Juntas1/1 -> Mux1/2
  Demux1/5 -> Modelo Juntas4/1
  Demux1/4 -> Modelo Juntas3/1
  Demux1/3 -> Modelo Juntas2/1
  Modelo Juntas2/1 -> Mux1/3
  Modelo Juntas3/1 -> Mux1/4
  Modelo Juntas4/1 -> Mux1/5

== system ControleFF_D_NL/Dinâmica do robô2/Modelo atrito ==
  note: z
  note: zdot
  Thetadot : Inport
  Abs : Abs
  Add : Sum  Inputs=+++
  Divide : Product  Inputs=*/*
  Integrator : Integrator
  Sigma0 : Gain  Gain=sigma0
  Sigma1 : Gain  Gain=sigma1
  Sigma2 : Gain  Gain=sigma2
  Sum : Sum  Inputs=|+-
  s_Thetadot : Subsystem
      settings: PortSchema="{\"entries\":[{\"content\":{\"sides\":[{\"content\":{\"connectorIds\":[]},\"type\":\"ConnectorPlacement.EquallySpacedRectSide\",\"uuid\":\"4c4b190b-c928-4253-93d1-fd2ae137e0ab\"},{\"content\":{\"connectorIds\":[\"Out1\"],\"side\":\"RIGHT\"},\"type\":\"ConnectorPlacement.EquallySpacedRectSide\",\"uuid\":\"6a4109ad-b0a7-44dc-94f8-84112378c3da\"},{\"content\":{\"connectorIds\":[\"In1\"],\"side\":\"TOP\"},\"type\":\"ConnectorPlacement.EquallySpacedRectSide\",\"uuid\":\"364d9b06-17df-4fa5-ae25-87ed6816814d\"},{\"content\":{\"connectorIds\":[],\"side\":\"HIDDEN\"},\"type\":\"ConnectorPlacement.EquallySpacedRectSide\",\"uuid\":\"e93aa933-b8be-40f2-a8c0-ee27516241e6\"}]},\"type\":\"ConnectorPlacement.EquallySpacedConnector\",\"uuid\":\"c598e9c2-b687-45ab-b3d0-f2b281a49fb7\"}],\"packageUris\":[\"http://schema.mathworks.com/mf0/Connector/R2020b\"],\"version\":\"1.0\"}"
  tal_F : Outport
  wires:
  Sigma0/1 -> Divide/3, Add/3
  Sigma1/1 -> Add/2
  Divide/1 -> Sum/2
  Abs/1 -> s_Thetadot/1(|Thetadot|), Divide/1
  s_Thetadot/1(s_Thetadot) -> Divide/2
  Sum/1 -> Sigma1/1, Integrator/1
  Thetadot/1 -> Sigma2/1, Sum/1, Abs/1
  Sigma2/1 -> Add/1
  Integrator/1 -> Sigma0/1
  Add/1 -> tal_F/1

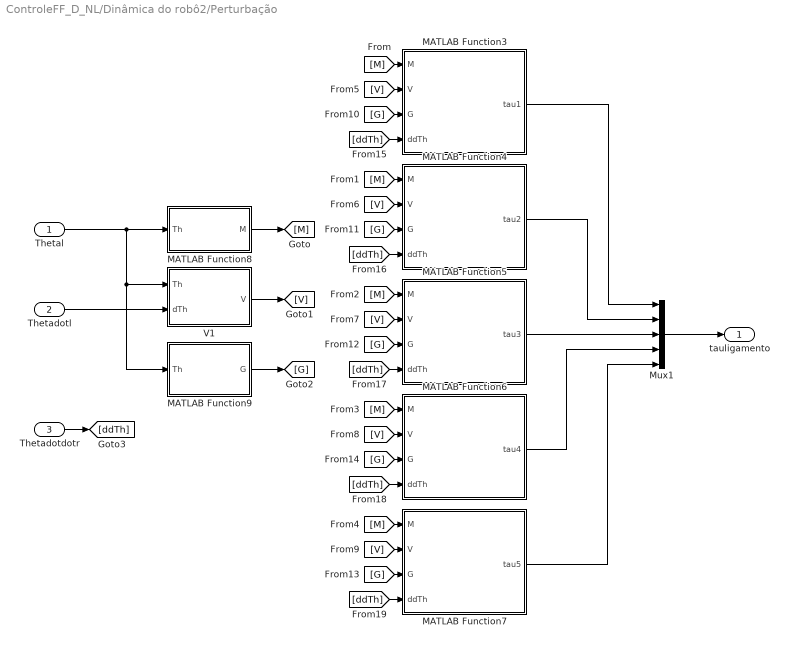
== system ControleFF_D_NL/Dinâmica do robô2/Perturbação ==
  Thetal : Inport
  Thetadotl : Inport  Port=2
  Thetadotdotr : Inport  Port=3
  MATLAB Function3 : MATLAB Function  TreatAsAtomicUnit=on
  MATLAB Function4 : MATLAB Function  TreatAsAtomicUnit=on
  MATLAB Function5 : MATLAB Function  TreatAsAtomicUnit=on
  MATLAB Function6 : MATLAB Function  TreatAsAtomicUnit=on
  MATLAB Function7 : MATLAB Function  TreatAsAtomicUnit=on
  MATLAB Function8 : MATLAB Function  TreatAsAtomicUnit=on
  MATLAB Function9 : MATLAB Function  TreatAsAtomicUnit=on
  Mux1 : Mux  Inputs=5
  V1 : MATLAB Function  TreatAsAtomicUnit=on
  tauligamento : Outport  VectorParamsAs1DForOutWhenUnconnected=off
  wires:
  [G] -> MATLAB Function6/3(G)
  MATLAB Function8/1(M) -> [M]
  [M] -> MATLAB Function6/1(M)
  [M] -> MATLAB Function4/1(M)
  [M] -> MATLAB Function3/1(M)
  Thetal/1 -> MATLAB Function8/1(Th), MATLAB Function9/1(Th), V1/1(Th)
  [ddTh] -> MATLAB Function5/4(ddTh)
  [V] -> MATLAB Function3/2(V)
  [ddTh] -> MATLAB Function3/4(ddTh)
  [G] -> MATLAB Function7/3(G)
  [ddTh] -> MATLAB Function6/4(ddTh)
  [V] -> MATLAB Function6/2(V)
  Thetadotl/1 -> V1/2(dTh)
  [G] -> MATLAB Function5/3(G)
  [G] -> MATLAB Function3/3(G)
  [G] -> MATLAB Function4/3(G)
  MATLAB Function9/1(G) -> [G]
  [V] -> MATLAB Function7/2(V)
  [ddTh] -> MATLAB Function4/4(ddTh)
  [V] -> MATLAB Function5/2(V)
  [V] -> MATLAB Function4/2(V)
  V1/1(V) -> [V]
  [M] -> MATLAB Function7/1(M)
  [M] -> MATLAB Function5/1(M)
  [ddTh] -> MATLAB Function7/4(ddTh)
  Mux1/1 -> tauligamento/1
  MATLAB Function3/1(tau1) -> Mux1/1
  MATLAB Function4/1(tau2) -> Mux1/2
  MATLAB Function5/1(tau3) -> Mux1/3
  MATLAB Function6/1(tau4) -> Mux1/4
  MATLAB Function7/1(tau5) -> Mux1/5
  Thetadotdotr/1 -> [ddTh]

== system ControleFF_D_NL/Compensador Feedforward/Modelo atrito/s_Thetadot ==
  |Thetadot| : Inport
  -alpha : Gain  Gain=-alpha
  Fc : Constant  Value=Fc
  Fs : Constant  Value=Fs
  Math Function : Math  SaturateOnIntegerOverflow=on
  Product : Product
  Sum1 : Sum  Inputs=|++
  Sum2 : Sum  Inputs=|-+
  s_Thetadot : Outport
  wires:
  |Thetadot|/1 -> -alpha/1
  Fc/1 -> Sum2/1, Sum1/2
  -alpha/1 -> Math Function/1
  Sum1/1 -> s_Thetadot/1
  Fs/1 -> Sum2/2
  Math Function/1 -> Product/1
  Sum2/1 -> Product/2
  Product/1 -> Sum1/1

== system ControleFF_D_NL/Dinâmica do robô/Modelo atrito/s_Thetadot ==
  |Thetadot| : Inport
  -alpha : Gain  Gain=-alpha
  Fc : Constant  Value=Fc
  Fs : Constant  Value=Fs
  Math Function : Math  SaturateOnIntegerOverflow=on
  Product : Product
  Sum1 : Sum  Inputs=|++
  Sum2 : Sum  Inputs=|-+
  s_Thetadot : Outport
  wires:
  |Thetadot|/1 -> -alpha/1
  Fc/1 -> Sum2/1, Sum1/2
  -alpha/1 -> Math Function/1
  Sum1/1 -> s_Thetadot/1
  Fs/1 -> Sum2/2
  Math Function/1 -> Product/1
  Sum2/1 -> Product/2
  Product/1 -> Sum1/1

== system ControleFF_D_NL/Dinâmica do robô2/Modelo atrito/s_Thetadot ==
  |Thetadot| : Inport
  -alpha : Gain  Gain=-alpha
  Fc : Constant  Value=Fc
  Fs : Constant  Value=Fs
  Math Function : Math  SaturateOnIntegerOverflow=on
  Product : Product
  Sum1 : Sum  Inputs=|++
  Sum2 : Sum  Inputs=|-+
  s_Thetadot : Outport
  wires:
  |Thetadot|/1 -> -alpha/1
  Fc/1 -> Sum2/1, Sum1/2
  -alpha/1 -> Math Function/1
  Sum1/1 -> s_Thetadot/1
  Fs/1 -> Sum2/2
  Math Function/1 -> Product/1
  Sum2/1 -> Product/2
  Product/1 -> Sum1/1

== matlab function ControleFF_D_NL/Dinâmica do robô1/Perturbação/MATLAB Function4 ==
  data: M input; V input; tau2 output; G input; ddTh input
function tau2  = calcul_dk2(M, V, G, ddTh)

tau2 = M(2,1)*ddTh(1) + M(2,3)*ddTh(3) + M(2,4)*ddTh(4) + M(2,5)*ddTh(5) ...
       + V(2) + G(2);

== matlab function ControleFF_D_NL/Dinâmica do robô1/Perturbação/MATLAB Function5 ==
  data: M input; V input; tau3 output; G input; ddTh input
function tau3  = calcul_dk3(M, V, G, ddTh)

tau3 = M(3,1)*ddTh(1) + M(3,2)*ddTh(2) + M(3,4)*ddTh(4) + M(3,5)*ddTh(5) ...
       + V(3) + G(3);

== matlab function ControleFF_D_NL/Dinâmica do robô1/Perturbação/MATLAB Function6 ==
  data: M input; V input; tau4 output; G input; ddTh input
function tau4 = calcul_dk4(M, V, G, ddTh)

tau4 = M(4,1)*ddTh(1) + M(4,2)*ddTh(2) + M(4,3)*ddTh(3) + M(4,5)*ddTh(5) ...
       + V(4) + G(4);

== matlab function ControleFF_D_NL/Dinâmica do robô1/Perturbação/MATLAB Function7 ==
  data: M input; V input; tau5 output; G input; ddTh input
function tau5  = calcul_dk5(M, V, G, ddTh)

tau5 = M(5,1)*ddTh(1) + M(5,2)*ddTh(2) + M(5,3)*ddTh(3) + M(5,4)*ddTh(4) ...
       + V(5) + G(5);
